simulink model "dsp_filter"  (R2026a)
settings: Solver=FixedStepDiscrete  StopTime=1200
values from neighbouring files (symbols this model uses):
  b_hp = [0.00301933028362 0.00496099322468 0.00667830481616 0 -0.0251916579703 -0.0720648094763 -0.130626662776 -0.180070826746 0.797892085297 -0.180070826746 -0.130626662776 -0.0720648094763 ... (17 elements, 1x17)]    [variables.mat]
  b_lp = [-0.00306200334634 -0.00503110836783 -0.00677269121763 0 0.025547698913 0.0730833221416 0.132472846946 0.182615819497 0.202292230868 0.182615819497 0.132472846946 0.0730833221416 ... (17 elements, 1x17)]    [variables.mat]
  SW0 = 0    [variables.mat]
  SW1 = 0    [variables.mat]
  SW2 = 0    [variables.mat]
libraries: dsphdlfiltering2 x2, dsphdlsigops2 x1
settings Model: DataTypeOverride=Off  Creator=KoayXianCong  LastModifiedBy=KoayXianCong
settings OptimizationCC: ConditionallyExecuteInputs=off  InheritOutputTypeSmallerThanSingle=on
settings DebuggingCC: ArtificialAlgebraicLoopMsg=error  SingleTaskRateTransMsg=error
settings HardwareCC: ProdHWDeviceType=ASIC/FPGA->ASIC/FPGA  TargetBitPerPointer=64.0  TargetBitPerSizeT=64.0  TargetBitPerPtrDiffT=64.0  TargetLongLongMode=on  TargetIntDivRoundTo=Zero  TargetEndianess=LittleEndian  TargetWordSize=64.0  TargetHWDeviceType=Custom Processor->MATLAB Host Computer  ProdEqTarget=off

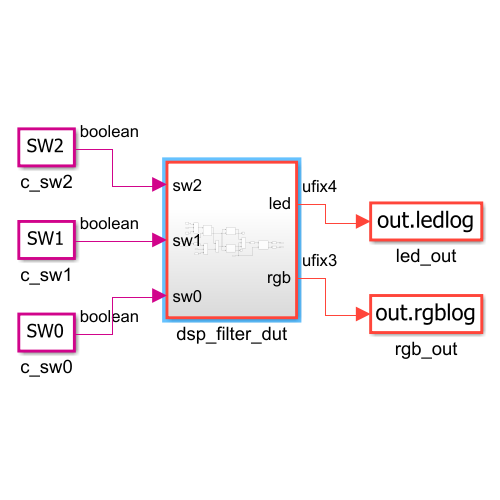
[thumbnail: Simulink's stored preview of the top-level diagram]
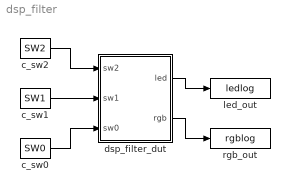
== system dsp_filter ==
  c_sw0 : Constant  Value=SW0  OutDataTypeStr=boolean
  c_sw1 : Constant  Value=SW1  OutDataTypeStr=boolean
  c_sw2 : Constant  Value=SW2  OutDataTypeStr=boolean
  dsp_filter_dut : Subsystem
  led_out : ToWorkspace  VariableName=ledlog  SaveFormat=Timeseries  SampleTime=-1
  rgb_out : ToWorkspace  VariableName=rgblog  SaveFormat=Timeseries  SampleTime=-1
  wires:
  c_sw2/1 -> dsp_filter_dut/1(sw2)
  c_sw1/1 -> dsp_filter_dut/2(sw1)
  c_sw0/1 -> dsp_filter_dut/3(sw0)
  dsp_filter_dut/1(led) -> led_out/1
  dsp_filter_dut/2(rgb) -> rgb_out/1

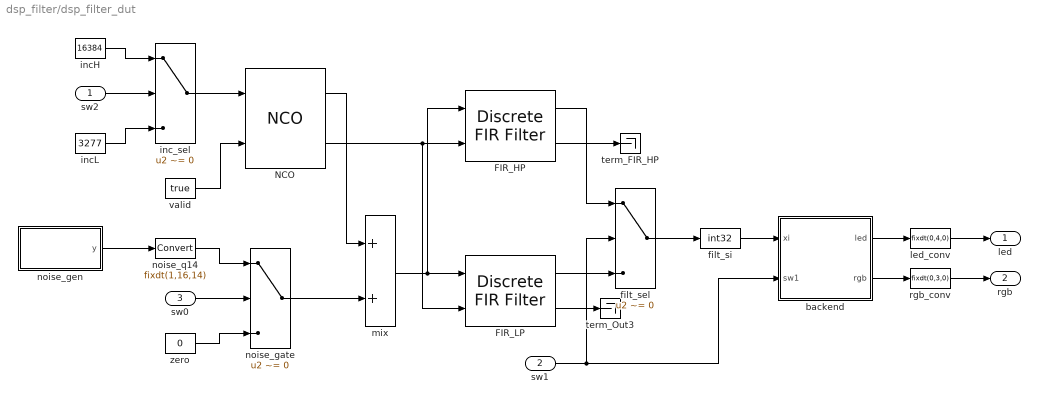
== system dsp_filter/dsp_filter_dut ==
  sw2 : Inport
  sw1 : Inport  Port=2
  sw0 : Inport  Port=3
  FIR_HP : dsphdlfiltering2/Discrete FIR Filter  NumeratorSource=Property  Numerator=b_hp  NumeratorPrototype=[]  FilterStructure=Direct form systolic  SerializationOption=Maximum number of multipliers  NumCycles=2  NumberOfMultipliers=17  SimulateUsing=Code generation  roundingMode=Floor  overflowMode=off  CoefficientsDataTypeStr=Inherit: Same word length as input  OutputDataTypeStr=fixdt(1,18,14)  ResetInputPort=off  HDLGlobalReset=off  CoeffMultiplier=Multiplier  UseMultForPow2Coeff=on  FrameInputSymmOptim=on
  FIR_LP : dsphdlfiltering2/Discrete FIR Filter  NumeratorSource=Property  Numerator=b_lp  NumeratorPrototype=[]  FilterStructure=Direct form systolic  SerializationOption=Maximum number of multipliers  NumCycles=2  NumberOfMultipliers=17  SimulateUsing=Code generation  roundingMode=Floor  overflowMode=off  CoefficientsDataTypeStr=Inherit: Same word length as input  OutputDataTypeStr=fixdt(1,18,14)  ResetInputPort=off  HDLGlobalReset=off  CoeffMultiplier=Multiplier  UseMultForPow2Coeff=on  FrameInputSymmOptim=on
  NCO : dsphdlsigops2/NCO  PhaseIncrementSource=Input port  PhaseIncrement=100  Frequency=510  FreqResolution=0.05  SamplingFreq=4000  PhaseOffsetSource=Property  PhaseOffset=0  PhaseOffsetR=pi/3  DitherSource=Property  NumDitherBits=4  SamplesPerFrame=1  LUTCompress=off  ResetAction=off  Waveform=Sine  PhasePort=off  SimulateUsing=Code generation  AccumulatorWL=16  PhaseQuantization=on  NumQuantizerAccumulatorBits=12  OutputDataType=Binary point scaling  OutputWL=16  OutputFL=14
      settings: LibrarySourceBlock=dsphdlsrcs2/NCO
  backend : MATLAB Function  TreatAsAtomicUnit=on
  filt_sel : Switch  Criteria=u2 ~= 0  SaturateOnIntegerOverflow=off  InputSameDT=off
  filt_si : DataTypeConversion  OutDataTypeStr=int32  ConvertRealWorld=Stored Integer (SI)  SaturateOnIntegerOverflow=off  RndMeth=Floor
  incH : Constant  Value=16384  OutDataTypeStr=fixdt(1,16,0)
  incL : Constant  Value=3277  OutDataTypeStr=fixdt(1,16,0)
  inc_sel : Switch  Criteria=u2 ~= 0  SaturateOnIntegerOverflow=off  InputSameDT=off
  led_conv : DataTypeConversion  OutDataTypeStr=fixdt(0,4,0)  SaturateOnIntegerOverflow=off  RndMeth=Floor
  mix : Sum  OutDataTypeStr=fixdt(1,16,14)
  noise_gate : Switch  Criteria=u2 ~= 0  SaturateOnIntegerOverflow=off  InputSameDT=off
  noise_gen : MATLAB Function  TreatAsAtomicUnit=on
  noise_q14 : DataTypeConversion  OutDataTypeStr=fixdt(1,16,14)  ConvertRealWorld=Stored Integer (SI)  SaturateOnIntegerOverflow=off  RndMeth=Floor
  rgb_conv : DataTypeConversion  OutDataTypeStr=fixdt(0,3,0)  SaturateOnIntegerOverflow=off  RndMeth=Floor
  term_FIR_HP : Terminator
  term_Out3 : Terminator
  valid : Constant  Value=true  OutDataTypeStr=boolean
  zero : Constant  Value=0  OutDataTypeStr=fixdt(1,16,14)
  led : Outport
  rgb : Outport  Port=2
  wires:
  noise_gen/1(y) -> noise_q14/1
  incH/1 -> inc_sel/1
  sw2/1 -> inc_sel/2
  incL/1 -> inc_sel/3
  inc_sel/1 -> NCO/1
  noise_q14/1 -> noise_gate/1
  sw0/1 -> noise_gate/2
  valid/1 -> NCO/2
  filt_si/1 -> backend/1(xi)
  zero/1 -> noise_gate/3
  NCO/2 -> FIR_HP/2, FIR_LP/2
  NCO/1 -> mix/1
  noise_gate/1 -> mix/2
  mix/1 -> FIR_LP/1, FIR_HP/1
  FIR_HP/1 -> filt_sel/1
  FIR_HP/2 -> term_FIR_HP/1
  FIR_LP/1 -> filt_sel/3
  sw1/1 -> backend/2(sw1), filt_sel/2
  filt_sel/1 -> filt_si/1
  backend/1(led) -> led_conv/1
  backend/2(rgb) -> rgb_conv/1
  led_conv/1 -> led/1
  rgb_conv/1 -> rgb/1
  FIR_LP/2 -> term_Out3/1

== matlab function dsp_filter/dsp_filter_dut/backend ==
  data: xi input; led output; sw1 input; rgb output
function [led, rgb] = backend(xi, sw1)
%#codegen - envelope detector + LED driver
% envelope tracking - measures how "strong" the signal is. ax = abs(xi) takes the magnitude (ignores whether the wave is above or below zero). 
  persistent e
  if isempty(e)
    e = int32(0);
  end
  ax = abs(xi);
  e = e + bitsra(ax - e, 6);
  % level bar - compares the envelope against four rising thresholds (1600 / 3500 / 5500 / 7500)
  b0 = e > int32(1600);
  b1 = e > int32(3500);
  b2 = e > int32(5500);
  b3 = e > int32(7500);
  led = uint8(b0) + uint8(b1)*uint8(2) + uint8(b2)*uint8(4) + uint8(b3)*uint8(8);
  % mode color -  sets the RGB LED based on the filter switch
  if sw1
    rgb = uint8(4);
  else
    rgb = uint8(2);
  end
end

== matlab function dsp_filter/dsp_filter_dut/noise_gen ==
  data: y output
function y = noise_gen()
%#codegen
  persistent state
  if isempty(state)
    state = uint16(44257);
  end
  lsb = bitand(state, uint16(1));
  state = bitshift(state, -1);
  if lsb == uint16(1)
    state = bitxor(state, uint16(46080));
  end
  hi = int16(bitshift(state, -8));
  y = hi*int16(64) - int16(8192);
end
